simulink model "cefasControl"  (R2020b)
settings: Solver=VariableStepAuto  StartTime=0.0  StopTime=2000  RelTol=1e-3
values from neighbouring files (symbols this model uses):
  den_ = modelTF.Denominator    [modelWork.m]
  denD = cell2mat(modelDiscrete.Denominator)    [modelWork.m]
  num_ = modelTF.Numerator    [modelWork.m]
  numD = cell2mat(modelDiscrete.Numerator)    [modelWork.m]
  Ts_ = mean(time(2:end)-time(1:end-1))    [modelWork.m]
libraries: pid_lib x2, fuzblock x1
settings Model: Creator=golam  LastModifiedBy=golam

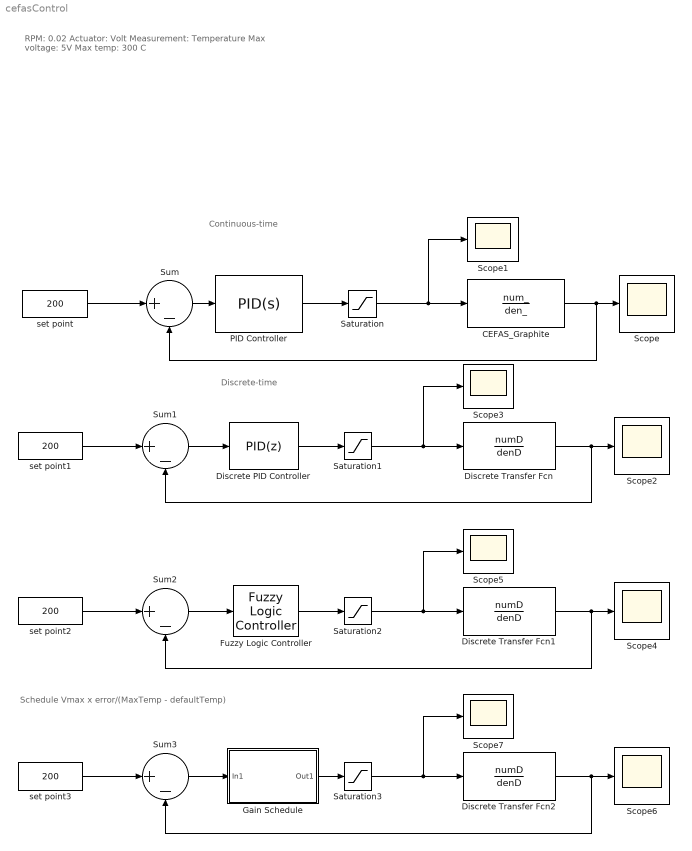
== system cefasControl ==
  note: Schedule
      |
      | Vmax x error/(MaxTemp - defaultTemp)
  note: Continuous-time
  note: RPM: 0.02
      |
      | Actuator: Volt
      | Measurement: Temperature
      |
      | Max voltage: 5V
      | Max temp: 300 C
  note: Discrete-time
  CEFAS_Graphite : TransferFcn  Numerator=num_  Denominator=den_
  Discrete Transfer Fcn : DiscreteTransferFcn  Numerator=numD  Denominator=denD  SampleTime=Ts_
  Discrete Transfer Fcn1 : DiscreteTransferFcn  Numerator=numD  Denominator=denD  SampleTime=Ts_
  Discrete Transfer Fcn2 : DiscreteTransferFcn  Numerator=numD  Denominator=denD  SampleTime=Ts_
  Discrete PID Controller : pid_lib/PID Controller  Controller=PID  Form=Parallel  TimeDomain=Discrete-time  UseExternalTs=off  SampleTime=Ts_  IntegratorMethod=Forward Euler  FilterMethod=Forward Euler  ControllerParametersSource=internal  P=0.0115212435203064  I=3.36670845921789e-05  D=0  UseFilter=on  N=100  TunerSelectOption=Transfer Function Based (PID Tuner App)  InitialConditionSource=internal  InitialConditionForIntegrator=0  InitialConditionForFilter=0  DifferentiatorICPrevScaledInput=0  ExternalReset=none  TrackingMode=off  Kt=1  LimitOutput=off  SatLimitsSource=internal  UpperSaturationLimit=inf  LowerSaturationLimit=-inf  LinearizeAsGain=off  AntiWindupMode=none  Kb=1  POutMin=[]  POutMax=[]  IOutMin=[]  IOutMax=[]  DOutMin=[]  DOutMax=[]  NOutMin=[]  NOutMax=[]  SumOutMin=[]  SumOutMax=[]  SaturationOutMin=[]  SaturationOutMax=[]  PParamMin=[]  PParamMax=[]  IParamMin=[]  IParamMax=[]  DParamMin=[]  DParamMax=[]  NParamMin=[]  NParamMax=[]  KbParamMin=[]  KbParamMax=[]  KtParamMin=[]  KtParamMax=[]  KbOutMin=[]  KbOutMax=[]  KtOutMin=[]  KtOutMax=[]  IntegratorOutMin=[]  IntegratorOutMax=[]  FilterOutMin=[]  FilterOutMax=[]  SumI1OutMin=[]  SumI1OutMax=[]  SumI2OutMin=[]  SumI2OutMax=[]  SumI3OutMin=[]  SumI3OutMax=[]  SumI4OutMin=[]  SumI4OutMax=[]  SumDOutMin=[]  SumDOutMax=[]  DifferentiatorOutMin=[]  DifferentiatorOutMax=[]  FilterDiffOutCoefMin=[]  FilterDiffOutCoefMax=[]  ReciprocalOutMin=[]  ReciprocalOutMax=[]  SumDenOutMin=[]  SumDenOutMax=[]  SumNumOutMin=[]  SumNumOutMax=[]  DivideOutMin=[]  DivideOutMax=[]  UdiffTsProdOutMin=[]  UdiffTsProdOutMax=[]  NTsProdOutMin=[]  NTsProdOutMax=[]  UintegralTsProdOutMin=[]  UintegralTsProdOutMax=[]  UngainTsProdOutMin=[]  UngainTsProdOutMax=[]  IntegratorContinuousStateAttributes=''  IntegratorStateMustResolveToSignalObject=off  IntegratorRTWStateStorageClass=Auto  FilterContinuousStateAttributes=''  FilterStateMustResolveToSignalObject=off  FilterRTWStateStorageClass=Auto  ParallelPVariant=InternalParameters  IdealPVariant=Disabled  IVariant=InternalParameters  DVariant=InternalParameters  IntegratorVariant=Discrete  SatVariant=Disabled  AWVariant=Passthrough  PCopyVariant=Disabled  TRVariant=Disabled  FdbkBlocksVariant=Forward  IdealPFdbkVariant=Disabled  SatFdbkVariant=Disabled  DerivativeFilterVariant=ForwardEulerFilter  NVariant=InternalParameters  NCopyVariant=Disabled  FilterICVariant=InternalICsFilter  IntegratorICVariant=InternalICs  ExternalResetVariant=Disabled  TRSumVariant=Passthrough  SumFdbkVariant=Disabled  SumVariant=Sum_PID  TsampFilterVariant=InternalTs  TsampNgainVariant=Passthrough  TsampIntegralVariant=Passthrough  ExternalSaturationOutDataTypeStr=Inherit: Same as second input
  Fuzzy Logic Controller : fuzblock/Fuzzy Logic  Controller  FIS='fuzzyCEFAS.fis'  OutputSampleNumber=101  DataType=double  FuzzifiedInputs=off  RuleFiringStrengths=off  RuleOutputs=off  AggregatedOutputs=off  SimulateUsing=Interpreted execution  OutOfRangeInputValueMessage=warning  NoRuleFiredMessage=warning  EmptyOutputFuzzySetMessage=warning
  Gain Schedule : Subsystem
  PID Controller : pid_lib/PID Controller  Controller=PID  Form=Parallel  TimeDomain=Continuous-time  UseExternalTs=off  SampleTime=-1  IntegratorMethod=Forward Euler  FilterMethod=Forward Euler  ControllerParametersSource=internal  P=0.0269070726852448  I=0.00010338380179242  D=0.275567234489223  UseFilter=on  N=0.0101276365715165  TunerSelectOption=Transfer Function Based (PID Tuner App)  InitialConditionSource=internal  InitialConditionForIntegrator=0  InitialConditionForFilter=0  DifferentiatorICPrevScaledInput=0  ExternalReset=none  TrackingMode=off  Kt=1  LimitOutput=off  SatLimitsSource=internal  UpperSaturationLimit=inf  LowerSaturationLimit=-inf  LinearizeAsGain=on  AntiWindupMode=none  Kb=1  POutMin=[]  POutMax=[]  IOutMin=[]  IOutMax=[]  DOutMin=[]  DOutMax=[]  NOutMin=[]  NOutMax=[]  SumOutMin=[]  SumOutMax=[]  SaturationOutMin=[]  SaturationOutMax=[]  PParamMin=[]  PParamMax=[]  IParamMin=[]  IParamMax=[]  DParamMin=[]  DParamMax=[]  NParamMin=[]  NParamMax=[]  KbParamMin=[]  KbParamMax=[]  KtParamMin=[]  KtParamMax=[]  KbOutMin=[]  KbOutMax=[]  KtOutMin=[]  KtOutMax=[]  IntegratorOutMin=[]  IntegratorOutMax=[]  FilterOutMin=[]  FilterOutMax=[]  SumI1OutMin=[]  SumI1OutMax=[]  SumI2OutMin=[]  SumI2OutMax=[]  SumI3OutMin=[]  SumI3OutMax=[]  SumI4OutMin=[]  SumI4OutMax=[]  SumDOutMin=[]  SumDOutMax=[]  DifferentiatorOutMin=[]  DifferentiatorOutMax=[]  FilterDiffOutCoefMin=[]  FilterDiffOutCoefMax=[]  ReciprocalOutMin=[]  ReciprocalOutMax=[]  SumDenOutMin=[]  SumDenOutMax=[]  SumNumOutMin=[]  SumNumOutMax=[]  DivideOutMin=[]  DivideOutMax=[]  UdiffTsProdOutMin=[]  UdiffTsProdOutMax=[]  NTsProdOutMin=[]  NTsProdOutMax=[]  UintegralTsProdOutMin=[]  UintegralTsProdOutMax=[]  UngainTsProdOutMin=[]  UngainTsProdOutMax=[]  IntegratorContinuousStateAttributes=''  IntegratorStateMustResolveToSignalObject=off  IntegratorRTWStateStorageClass=Auto  FilterContinuousStateAttributes=''  FilterStateMustResolveToSignalObject=off  FilterRTWStateStorageClass=Auto  ParallelPVariant=InternalParameters  IdealPVariant=Disabled  IVariant=InternalParameters  DVariant=InternalParameters  IntegratorVariant=Continuous  SatVariant=Disabled  AWVariant=Passthrough  PCopyVariant=Disabled  TRVariant=Disabled  FdbkBlocksVariant=Forward  IdealPFdbkVariant=Disabled  SatFdbkVariant=Disabled  DerivativeFilterVariant=ContFilter  NVariant=InternalParameters  NCopyVariant=Disabled  FilterICVariant=InternalICsFilter  IntegratorICVariant=InternalICs  ExternalResetVariant=Disabled  TRSumVariant=Passthrough  SumFdbkVariant=Disabled  SumVariant=Sum_PID  TsampFilterVariant=InternalTs  TsampNgainVariant=Passthrough  TsampIntegralVariant=Passthrough  ExternalSaturationOutDataTypeStr=Inherit: Same as second input
  Saturation{,1..3} (4 alike) : Saturate  UpperLimit=4  LowerLimit=0
  Scope{,1..7} (8 alike) : Scope
  Sum{,1..3} (4 alike) : Sum  Inputs=|+-
  set point : Constant  Value=200
  set point1 : Constant  Value=200  SampleTime=Ts_
  set point2 : Constant  Value=200  SampleTime=Ts_
  set point3 : Constant  Value=200  SampleTime=Ts_
  wires:
  CEFAS_Graphite/1 -> Sum/2, Scope/1
  set point/1 -> Sum/1
  Sum/1 -> PID Controller/1
  PID Controller/1 -> Saturation/1
  Saturation/1 -> Scope1/1, CEFAS_Graphite/1
  Discrete PID Controller/1 -> Saturation1/1
  Sum1/1 -> Discrete PID Controller/1
  Saturation1/1 -> Scope3/1, Discrete Transfer Fcn/1
  set point1/1 -> Sum1/1
  Discrete Transfer Fcn/1 -> Sum1/2, Scope2/1
  Sum2/1 -> Fuzzy Logic Controller/1
  Saturation2/1 -> Scope5/1, Discrete Transfer Fcn1/1
  set point2/1 -> Sum2/1
  Fuzzy Logic Controller/1 -> Saturation2/1
  Discrete Transfer Fcn1/1 -> Sum2/2, Scope4/1
  Saturation3/1 -> Scope7/1, Discrete Transfer Fcn2/1
  set point3/1 -> Sum3/1
  Discrete Transfer Fcn2/1 -> Sum3/2, Scope6/1
  Sum3/1 -> Gain Schedule/1(In1)
  Gain Schedule/1(Out1) -> Saturation3/1

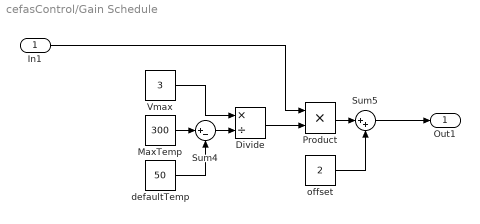
== system cefasControl/Gain Schedule ==
  In1 : Inport
  Divide : Product  Inputs=*/
  MaxTemp : Constant  Value=300  SampleTime=Ts_
  Product : Product
  Sum4 : Sum  Inputs=|+-
  Sum5 : Sum  Inputs=|++
  Vmax : Constant  Value=3  SampleTime=Ts_
  defaultTemp : Constant  Value=50  SampleTime=Ts_
  offset : Constant  Value=2
  Out1 : Outport
  wires:
  defaultTemp/1 -> Sum4/2
  In1/1 -> Product/1
  Sum4/1 -> Divide/2
  Divide/1 -> Product/2
  Product/1 -> Sum5/1
  Sum5/1 -> Out1/1
  Vmax/1 -> Divide/1
  MaxTemp/1 -> Sum4/1
  offset/1 -> Sum5/2
